simulink model "zadnanienr1_Simulink"  (R2024b)
settings: Solver=ode4  StartTime=0.0  StopTime=10.0  FixedStep=0.001  RelTol=1e-3
model workspace (MAT data in the model file):
  a = 1
  b = 1
  theta = 2
undefined symbols (not defined in the file or in its folder): k, licz, licz_new, mian, mian_new, T
settings Model: Creator=adasf  LastModifiedBy=adasf

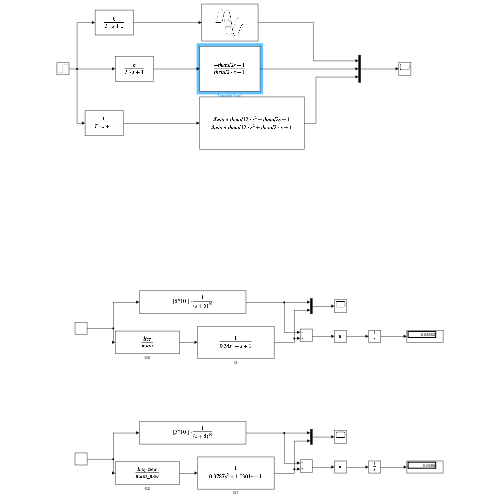
[thumbnail: Simulink's stored preview of the top-level diagram]
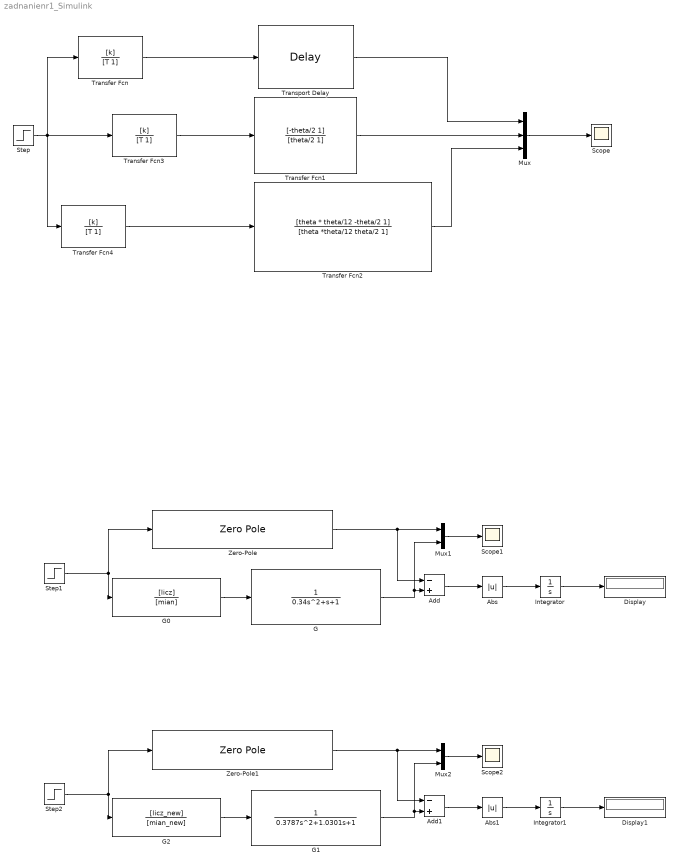
== system zadnanienr1_Simulink ==
  Abs : Abs  SaturateOnIntegerOverflow=off
  Abs1 : Abs  SaturateOnIntegerOverflow=off
  Add : Sum  Inputs=-+
  Add1 : Sum  Inputs=-+
  Display : Display
  Display1 : Display
  G : TransferFcn  Denominator=[0.34 1 1]
  G0 : TransferFcn  Numerator=[licz]  Denominator=[mian]
  G1 : TransferFcn  Denominator=[0.3787 1.0301 1]
  G2 : TransferFcn  Numerator=[licz_new]  Denominator=[mian_new]
  Integrator : Integrator
  Integrator1 : Integrator
  Mux : Mux  Inputs=3
  Mux1 : Mux  Inputs=2
  Mux2 : Mux  Inputs=2
  Scope : Scope
  Scope1 : Scope
  Scope2 : Scope
  Step : Step  Time=0  SampleTime=0
  Step1 : Step  SampleTime=0
  Step2 : Step  SampleTime=0
  Transfer Fcn : TransferFcn  Numerator=[k]  Denominator=[T 1]
  Transfer Fcn1 : TransferFcn  Numerator=[-theta/2 1]  Denominator=[theta/2 1]
  Transfer Fcn2 : TransferFcn  Numerator=[theta * theta/12 -theta/2 1]  Denominator=[theta *theta/12 theta/2 1]
  Transfer Fcn3 : TransferFcn  Numerator=[k]  Denominator=[T 1]
  Transfer Fcn4 : TransferFcn  Numerator=[k]  Denominator=[T 1]
  Transport Delay : TransportDelay  DelayTime=theta
  Zero-Pole : ZeroPole  Zeros=[]  Poles=[-5 -5 -5 -5 -5 -5 -5 -5 -5 -5]  Gain=[5^10]
  Zero-Pole1 : ZeroPole  Zeros=[]  Poles=[-5 -5 -5 -5 -5 -5 -5 -5 -5 -5]  Gain=[5^10]
  wires:
  Transfer Fcn1/1 -> Mux/2
  Transport Delay/1 -> Mux/1
  Mux/1 -> Scope/1
  Transfer Fcn3/1 -> Transfer Fcn1/1
  Transfer Fcn4/1 -> Transfer Fcn2/1
  Transfer Fcn/1 -> Transport Delay/1
  Step/1 -> Transfer Fcn4/1, Transfer Fcn3/1, Transfer Fcn/1
  G0/1 -> G/1
  Step1/1 -> G0/1, Zero-Pole/1
  G/1 -> Mux1/2, Add/2
  Zero-Pole/1 -> Add/1, Mux1/1
  Mux1/1 -> Scope1/1
  Add/1 -> Abs/1
  Integrator/1 -> Display/1
  Abs/1 -> Integrator/1
  G1/1 -> Mux2/2, Add1/2
  Integrator1/1 -> Display1/1
  Mux2/1 -> Scope2/1
  Zero-Pole1/1 -> Add1/1, Mux2/1
  Add1/1 -> Abs1/1
  Abs1/1 -> Integrator1/1
  Step2/1 -> G2/1, Zero-Pole1/1
  G2/1 -> G1/1
  Transfer Fcn2/1 -> Mux/3
